simulink model "user_sim"  (R2018a)
settings: Solver=VariableStepAuto  StartTime=0.0  StopTime=50  RelTol=1e-3
settings Model: Creator=mutou  LastModifiedBy=mutou

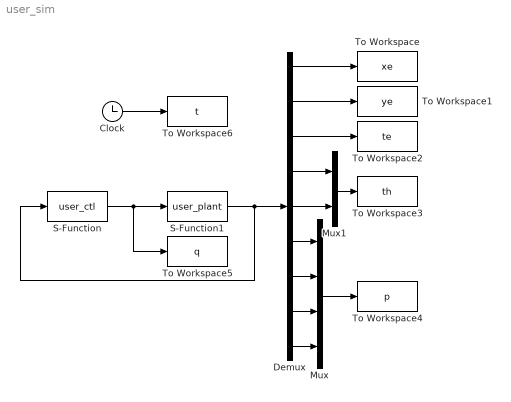
== system user_sim ==
  Clock : Clock
      settings: Decimation=50
  Demux : Demux  Outputs=9
  Mux : Mux
  Mux1 : Mux  Inputs=2
  S-Function : S-Function  FunctionName=user_ctl  SFunctionDeploymentMode=off  EnableBusSupport=off
  S-Function1 : S-Function  FunctionName=user_plant  SFunctionDeploymentMode=off  EnableBusSupport=off
  To Workspace : ToWorkspace  VariableName=xe  SampleTime=-1
  To Workspace1 : ToWorkspace  VariableName=ye  SampleTime=-1
  To Workspace2 : ToWorkspace  VariableName=te  SampleTime=-1
  To Workspace3 : ToWorkspace  VariableName=th  SampleTime=-1
  To Workspace4 : ToWorkspace  VariableName=p  SampleTime=-1
  To Workspace5 : ToWorkspace  VariableName=q  SampleTime=-1
  To Workspace6 : ToWorkspace  VariableName=t  SampleTime=-1
  wires:
  Mux/1 -> To Workspace4/1
  Demux/1 -> To Workspace/1
  Demux/2 -> To Workspace1/1
  Demux/3 -> To Workspace2/1
  Mux1/1 -> To Workspace3/1
  S-Function1/1 -> S-Function/1, Demux/1
  S-Function/1 -> To Workspace5/1, S-Function1/1
  Clock/1 -> To Workspace6/1
  Demux/4 -> Mux1/1
  Demux/5 -> Mux1/2
  Demux/6 -> Mux/1
  Demux/7 -> Mux/2
  Demux/8 -> Mux/3
  Demux/9 -> Mux/4
